simulink model "sedemo_star_routing"  (Simulink 7.5)
settings: Solver=VariableStepDiscrete  StartTime=0.0  StopTime=100  MaxStep=inf  RelTol=1e-3
undefined symbols (not defined in the file or in its folder): des_attributefunction_support
libraries: simeventsattributes2 x13, simeventssink1 x6, simeventsserver1 x5, simeventsrouting1 x4, simeventsgenerators1 x3, simeventstranslate1 x2, simeventsinfo x1
settings Model: Creator=The MathWorks Inc.  ExtModeAutoUpdateStatusClock=off
settings DataIOCC: SaveOutput=off  SignalLogging=off  SaveTime=off
settings OptimizationCC: InlineParams=on  InitFltsAndDblsToZero=on
settings DebuggingCC: AlgebraicLoopMsg=error  SolverPrmCheckMsg=none  StrictBusMsg=Warning
settings SimEventsCC: propDiagAttribOutput=1  propDiagFcnCallOutput=1  propDiagStatOutput=0

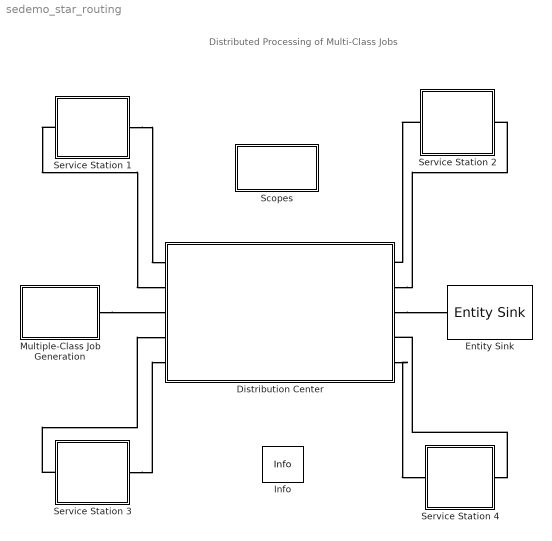
== system sedemo_star_routing ==
  note: Distributed Processing of Multi-Class Jobs
  Distribution Center : Subsystem  mask(Distribution Center){JobIDInWatch=1, RoutingDelay=.3}
      mask prompts: JobIDInWatch "Display service history for jobs with ID:"; RoutingDelay "Time needed for routing:"
      mask help:
      | Distribution center receives jobs from the source or remote service stations. It routes the job to its next service station based on job class and job service status.
      | Specify the time required for routing and the job ID that the service history monitor is tracing.
      mask Display:
      | color('blue')
      | fprintf('JOB ID: %s\n\nDouble Click to \nSelect Job ID.', get_param(gcb,'JobIDInWatch'))
  Entity Sink : simeventssink1/Entity Sink  Priority=1  SystemSampleTime=-1  AvailableForArrivals=on  StatNumberArrived=Off
  Info : simeventsinfo/Info  SystemSampleTime=-1
  Multiple-Class Job Generation : Subsystem
  Scopes : Subsystem
      mask Display: fprintf('Scopes')
  Service Station 1 : Subsystem
  Service Station 2 : Subsystem
  Service Station 3 : Subsystem
  Service Station 4 : Subsystem
  connections:
  Service Station 1/LConn1 -- Distribution Center/LConn2
  Distribution Center/RConn2 -- Service Station 2/LConn1
  Distribution Center/RConn5 -- Service Station 4/LConn1
  Service Station 3/LConn1 -- Distribution Center/LConn5
  Multiple-Class Job Generation/RConn1 -- Distribution Center/LConn3
  Distribution Center/RConn3 -- Entity Sink/LConn1
  Service Station 2/RConn1 -- Distribution Center/RConn1
  Service Station 1/RConn1 -- Distribution Center/LConn1
  Service Station 3/RConn1 -- Distribution Center/LConn4
  Service Station 4/RConn1 -- Distribution Center/RConn4

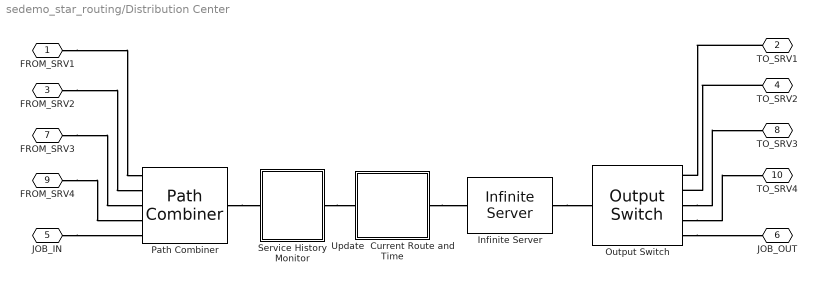
== system sedemo_star_routing/Distribution Center ==
  Infinite Server : simeventsserver1/Infinite Server  Priority=1  SystemSampleTime=-1  ServiceTimeFrom=Dialog  ServiceTime=RoutingDelay  AttributeName=ServiceTime  PriorityServiceCompletion=5  EnableTOPort=off  StatNumberDeparted=Off  StatNumberInBlock=Off  StatPendingEntity=Off  StatNumberPending=Off  StatAverageWait=Off  StatNumberTimedout=Off
  Output Switch : simeventsrouting1/Output Switch  Priority=1  SystemSampleTime=-1  NumberOutputPorts=5  SwitchingCriterion=From attribute  InitialSeed=34567  AttributeName=CurrentRoute  InitialConditionsOpt=off  InitialConditions=1  EntityBufferOpt=off  SpecifyEventPriority=off  PriorityOutputSwitchSelectPort=4100  TimeoutPortOpt=off  StatNumberDeparted=Off  StatNumberTimedOut=Off  StatPendingEntity=Off  StatLastDeparturePort=Off  EvaluatedNumPorts=5
  Path Combiner : simeventsrouting1/Path Combiner  Priority=1  SystemSampleTime=-1  NumberInputPorts=5  InputPortPrecedence=IN1 port  InitialSeed=45675  SpecifyEventPriority=off  PriorityPathCombinerPortPrecedenceSelection=4100  StatNumberDeparted=Off  StatLastArrivalPort=Off  EvaluatedNumPorts=5
  Service History Monitor : Subsystem
  Update  Current Route and Time : Subsystem  LoadFcn=des_attributefunction_support(gcb,'LoadFcn');  StartFcn=des_attributefunction_support(gcb,'StartFcn');  mask(Attribute Function){OutputNamePrefix=out_}
      mask prompts: OutputNamePrefix "Prefix name"
      settings: CopyFcn=des_attributefunction_support(gcb,'CopyFcn');  OpenFcn=des_attributefunction_support(gcb,'OpenFcn');  ErrorFcn=des_error_redirect
      mask Display: image(des_iconLoad('attribFunction.jpg'),'center');
  FROM_SRV1 : PMIOPort  Port=1  Side=Left
  TO_SRV1 : PMIOPort  Port=2  Side=Left
  FROM_SRV2 : PMIOPort  Port=3  Side=Right
  TO_SRV2 : PMIOPort  Port=4  Side=Right
  JOB_IN : PMIOPort  Port=5  Side=Left
  JOB_OUT : PMIOPort  Port=6  Side=Right
  FROM_SRV3 : PMIOPort  Port=7  Side=Left
  TO_SRV3 : PMIOPort  Port=8  Side=Left
  FROM_SRV4 : PMIOPort  Port=9  Side=Right
  TO_SRV4 : PMIOPort  Port=10  Side=Right
  connections:
  TO_SRV1/RConn1 -- Output Switch/RConn1
  FROM_SRV1/RConn1 -- Path Combiner/LConn1
  TO_SRV2/RConn1 -- Output Switch/RConn2
  FROM_SRV2/RConn1 -- Path Combiner/LConn2
  Output Switch/RConn3 -- TO_SRV3/RConn1
  Output Switch/RConn4 -- TO_SRV4/RConn1
  Output Switch/RConn5 -- JOB_OUT/RConn1
  FROM_SRV3/RConn1 -- Path Combiner/LConn3
  FROM_SRV4/RConn1 -- Path Combiner/LConn4
  JOB_IN/RConn1 -- Path Combiner/LConn5
  Path Combiner/RConn1 -- Service History Monitor/LConn1
  Update  Current Route and Time/RConn1 -- Infinite Server/LConn1
  Infinite Server/RConn1 -- Output Switch/LConn1
  Service History Monitor/RConn1 -- Update  Current Route and Time/LConn1

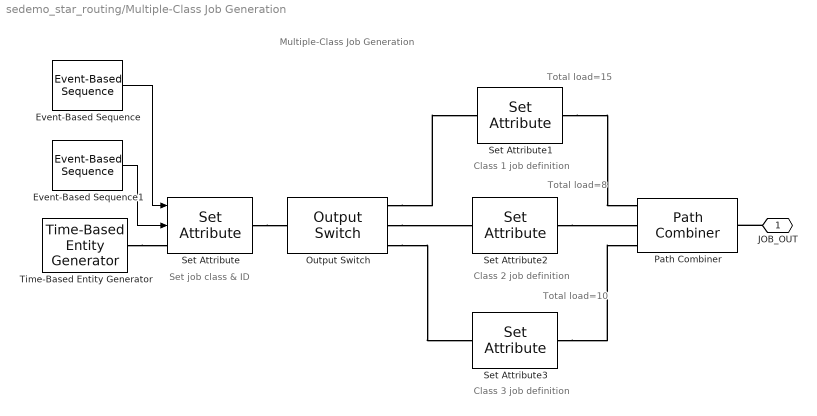
== system sedemo_star_routing/Multiple-Class Job Generation ==
  note: Set job class & ID
  note: Class 1 job definition
  note: Class 2 job definition
  note: Class 3 job definition
  note: Total load=15
  note: Total load=8
  note: Total load=10
  note: Multiple-Class Job Generation
  Event-Based Sequence : simeventsgenerators1/Signal Generators/Event-Based Sequence  SystemSampleTime=-1  VectorOutputValues=1:3  FormOutputOpt=Cyclic repetition  IsProcessed=on  isConnected=1
  Event-Based Sequence1 : simeventsgenerators1/Signal Generators/Event-Based Sequence  SystemSampleTime=-1  VectorOutputValues=1:15  FormOutputOpt=Cyclic repetition  IsProcessed=on  isConnected=1
  Output Switch : simeventsrouting1/Output Switch  Priority=1  SystemSampleTime=-1  NumberOutputPorts=3  SwitchingCriterion=From attribute  InitialSeed=34567  AttributeName=JobClass  InitialConditionsOpt=off  InitialConditions=1  EntityBufferOpt=off  SpecifyEventPriority=off  PriorityOutputSwitchSelectPort=4100  TimeoutPortOpt=off  StatNumberDeparted=Off  StatNumberTimedOut=Off  StatPendingEntity=Off  StatLastDeparturePort=Off  EvaluatedNumPorts=3
  Path Combiner : simeventsrouting1/Path Combiner  Priority=1  SystemSampleTime=-1  NumberInputPorts=3  InputPortPrecedence=IN1 port  InitialSeed=45675  SpecifyEventPriority=off  PriorityPathCombinerPortPrecedenceSelection=4100  StatNumberDeparted=Off  StatLastArrivalPort=Off  EvaluatedNumPorts=3
  Set Attribute : simeventsattributes2/Set Attribute  Priority=1  DialogController=des_ddg_create  DialogControllerArgs=DataTag19  SystemSampleTime=-1  AttributeFrom=Signal port|Signal port|Dialog|Dialog  AttributeName=JobClass|JobID|LastServiceLocation|JobServiceStatus  AttributeTreatAsVector=1|1|1|0  AttributeValue=1|1|0|zeros(1,15)  AttributeCreate=on  StatNumberDeparted=Off  EvaluatedAttributeValue={1}
  Set Attribute1 : simeventsattributes2/Set Attribute  Priority=1  DialogController=des_ddg_create  DialogControllerArgs=DataTag21  SystemSampleTime=-1  AttributeFrom=Dialog|Dialog|Dialog  AttributeName=ServiceProcess|ServiceTime|CurrentStep  AttributeTreatAsVector=1|1|1  AttributeValue=[1 2 4 2 3 5]|[2 1 5 3 4 0]|1  AttributeCreate=on  StatNumberDeparted=Off  EvaluatedAttributeValue={1}
  Set Attribute2 : simeventsattributes2/Set Attribute  Priority=1  DialogController=des_ddg_create  DialogControllerArgs=DataTag23  SystemSampleTime=-1  AttributeFrom=Dialog|Dialog|Dialog  AttributeName=ServiceProcess|ServiceTime|CurrentStep  AttributeTreatAsVector=1|1|1  AttributeValue=[2 1 3 1 4 5]|[1 1 2 1 3 0]|1  AttributeCreate=on  StatNumberDeparted=Off  EvaluatedAttributeValue={1}
  Set Attribute3 : simeventsattributes2/Set Attribute  Priority=1  DialogController=des_ddg_create  DialogControllerArgs=DataTag25  SystemSampleTime=-1  AttributeFrom=Dialog|Dialog|Dialog  AttributeName=ServiceProcess|ServiceTime|CurrentStep  AttributeTreatAsVector=1|1|1  AttributeValue=[4 2 1 2 3 5]|[5 1 2 1 1 0]|1  AttributeCreate=on  StatNumberDeparted=Off  EvaluatedAttributeValue={1}
  Time-Based Entity Generator : simeventsgenerators1/Entity Generators/Time-Based Entity Generator  Priority=1  DialogController=des_ddg_create  DialogControllerArgs=DataTag27  SystemSampleTime=-1  GenerateEntitiesUpon=Intergeneration time from dialog  Distribution=Uniform  Minimum=1  Maximum=2  Mean=1  InitialSeed=12345  Period=1  PriorityEntityGeneration=600  GenerateEntityAtSimulationStart=on  ResponseWhenBlocked=Pause generation  ResponseWhenUnblocked=Immediate restart  EntityType=Blank  StatNumberDeparted=Off  StatPendingEntity=Off  StatAverageIntergenerationTime=Off
  JOB_OUT : PMIOPort  Port=1  Side=Right
  wires:
  Event-Based Sequence/1 -> Set Attribute/1
  Event-Based Sequence1/1 -> Set Attribute/2
  connections:
  Set Attribute/RConn1 -- Output Switch/LConn1
  Output Switch/RConn1 -- Set Attribute1/LConn1
  Output Switch/RConn2 -- Set Attribute2/LConn1
  Output Switch/RConn3 -- Set Attribute3/LConn1
  Set Attribute1/RConn1 -- Path Combiner/LConn1
  Set Attribute2/RConn1 -- Path Combiner/LConn2
  Set Attribute3/RConn1 -- Path Combiner/LConn3
  Time-Based Entity Generator/RConn1 -- Set Attribute/LConn1
  JOB_OUT/RConn1 -- Path Combiner/RConn1

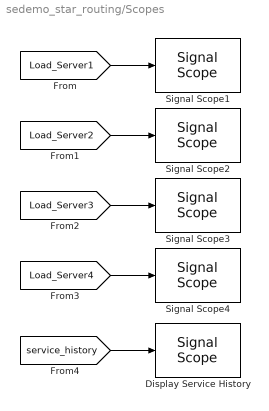
== system sedemo_star_routing/Scopes ==
  Display Service History : simeventssink1/Signal Scope  Priority=1  SystemSampleTime=-1  PlotType=Stair  InputType=Signal  NumInputs=1  AttributeNameY=Count  XInputOptionSignal=Event time  XInputOptionEntity=Event time  AttributeNameX=Count  EnableEntityOutport=on  XMin=0  XMax=110  XLimitExceededOption=Keep axis limits unchanged  YLimitExceededOption=Keep axis limits unchanged  AxisGrid=on  AxisLegend=off  LineDisables=""  LineColors="0  0  1"  LineStyles=-  LineMarkers=None  OpenScopeAtSimStart=on  Title=Service History for Jobs with Specified ID  YLabel=Service Station Visited  XLabel=Time  FigurePosition=[7 687 320 160]  AxisZoom=off  DataStoreOption=Limited  DataPointsLimit=10000  StatNumberArrived=Off  ShowCountPlotted=off  ShowToolbar=off
      settings: YMin=0  YMax=5
  Signal Scope1 : simeventssink1/Signal Scope  Priority=1  SystemSampleTime=-1  PlotType=Stair  InputType=Signal  NumInputs=1  AttributeNameY=Count  XInputOptionSignal=Event time  XInputOptionEntity=Event time  AttributeNameX=Count  EnableEntityOutport=on  XMin=0  XMax=10  XLimitExceededOption=Stretch axis limits  YLimitExceededOption=Stretch axis limits  AxisGrid=on  AxisLegend=off  LineDisables=""  LineColors="0  0  1"  LineStyles=-  LineMarkers=.  OpenScopeAtSimStart=on  Title=Load of Service Station 1  YLabel=Load  XLabel=Time  FigurePosition=[6 499 314 139]  AxisZoom=off  DataStoreOption=Limited  DataPointsLimit=10000  StatNumberArrived=Off  ShowCountPlotted=off  ShowToolbar=off
      settings: YMin=0  YMax=6
  Signal Scope2 : simeventssink1/Signal Scope  Priority=1  SystemSampleTime=-1  PlotType=Stair  InputType=Signal  NumInputs=1  AttributeNameY=Count  XInputOptionSignal=Event time  XInputOptionEntity=Event time  AttributeNameX=Count  EnableEntityOutport=on  XMin=0  XMax=10  XLimitExceededOption=Stretch axis limits  YLimitExceededOption=Stretch axis limits  AxisGrid=on  AxisLegend=off  LineDisables=""  LineColors="1  0  1"  LineStyles=-  LineMarkers=.  OpenScopeAtSimStart=on  Title=Load of Service Station 2  YLabel=Load  XLabel=Time  FigurePosition=[328 499 314 140]  AxisZoom=off  DataStoreOption=Limited  DataPointsLimit=10000  StatNumberArrived=Off  ShowCountPlotted=off  ShowToolbar=off
      settings: YMin=0  YMax=6
  Signal Scope3 : simeventssink1/Signal Scope  Priority=1  SystemSampleTime=-1  PlotType=Stair  InputType=Signal  NumInputs=1  AttributeNameY=Count  XInputOptionSignal=Event time  XInputOptionEntity=Event time  AttributeNameX=Count  EnableEntityOutport=on  XMin=0  XMax=10  XLimitExceededOption=Stretch axis limits  YLimitExceededOption=Stretch axis limits  AxisGrid=on  AxisLegend=off  LineDisables=""  LineColors="0  1  0"  LineStyles=-  LineMarkers=.  OpenScopeAtSimStart=on  Title=Load of Service Station 3  YLabel=Load  XLabel=Time  FigurePosition=[5 314 314 137]  AxisZoom=off  DataStoreOption=Limited  DataPointsLimit=10000  StatNumberArrived=Off  ShowCountPlotted=off  ShowToolbar=off
      settings: YMin=0  YMax=6
  Signal Scope4 : simeventssink1/Signal Scope  Priority=1  SystemSampleTime=-1  PlotType=Stair  InputType=Signal  NumInputs=1  AttributeNameY=Count  XInputOptionSignal=Event time  XInputOptionEntity=Event time  AttributeNameX=Count  EnableEntityOutport=on  XMin=0  XMax=10  XLimitExceededOption=Stretch axis limits  YLimitExceededOption=Stretch axis limits  AxisGrid=on  AxisLegend=off  LineDisables=""  LineColors="1  0  0"  LineStyles=-  LineMarkers=.  OpenScopeAtSimStart=on  Title=Load of Service Station 4  YLabel=Load  XLabel=Time  FigurePosition=[328 316 318 134]  AxisZoom=off  DataStoreOption=Limited  DataPointsLimit=10000  StatNumberArrived=Off  ShowCountPlotted=off  ShowToolbar=off
      settings: YMin=0  YMax=6
  wires:
  [Load_Server1] -> Signal Scope1/1
  [Load_Server4] -> Signal Scope4/1
  [Load_Server3] -> Signal Scope3/1
  [Load_Server2] -> Signal Scope2/1
  [service_history] -> Display Service History/1

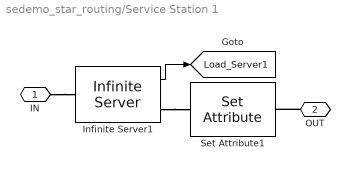
== system sedemo_star_routing/Service Station 1 ==
  Infinite Server1 : simeventsserver1/Infinite Server  Priority=1  SystemSampleTime=-1  ServiceTimeFrom=Attribute  ServiceTime=1  AttributeName=CurrentServiceTime  PriorityServiceCompletion=500  EnableTOPort=off  StatNumberDeparted=Off  StatNumberInBlock=On  StatPendingEntity=Off  StatNumberPending=Off  StatAverageWait=Off  StatNumberTimedout=Off
  Set Attribute1 : simeventsattributes2/Set Attribute  Priority=1  DialogController=des_ddg_create  DialogControllerArgs=DataTag35  SystemSampleTime=-1  AttributeFrom=Dialog  AttributeName=LastServiceLocation  AttributeTreatAsVector=1  AttributeValue=1  AttributeCreate=on  StatNumberDeparted=Off  EvaluatedAttributeValue={1}
  IN : PMIOPort  Port=1  Side=Left
  OUT : PMIOPort  Port=2  Side=Right
  tag scope: Load_Server1=global
  wires:
  Infinite Server1/1 -> [Load_Server1]
  connections:
  Infinite Server1/RConn1 -- Set Attribute1/LConn1
  IN/RConn1 -- Infinite Server1/LConn1
  OUT/RConn1 -- Set Attribute1/RConn1

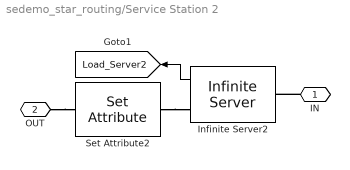
== system sedemo_star_routing/Service Station 2 ==
  Infinite Server2 : simeventsserver1/Infinite Server  Priority=1  SystemSampleTime=-1  ServiceTimeFrom=Attribute  ServiceTime=1  AttributeName=CurrentServiceTime  PriorityServiceCompletion=500  EnableTOPort=off  StatNumberDeparted=Off  StatNumberInBlock=On  StatPendingEntity=Off  StatNumberPending=Off  StatAverageWait=Off  StatNumberTimedout=Off
  Set Attribute2 : simeventsattributes2/Set Attribute  Priority=1  DialogController=des_ddg_create  DialogControllerArgs=DataTag38  SystemSampleTime=-1  AttributeFrom=Dialog  AttributeName=LastServiceLocation  AttributeTreatAsVector=1  AttributeValue=2  AttributeCreate=on  StatNumberDeparted=Off  EvaluatedAttributeValue={2}
  IN : PMIOPort  Port=1  Side=Left
  OUT : PMIOPort  Port=2  Side=Right
  tag scope: Load_Server2=global
  wires:
  Infinite Server2/1 -> [Load_Server2]
  connections:
  Set Attribute2/LConn1 -- Infinite Server2/RConn1
  IN/RConn1 -- Infinite Server2/LConn1
  OUT/RConn1 -- Set Attribute2/RConn1

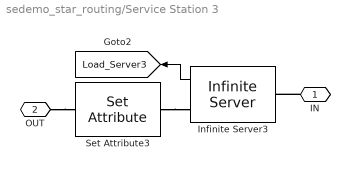
== system sedemo_star_routing/Service Station 3 ==
  Infinite Server3 : simeventsserver1/Infinite Server  Priority=1  SystemSampleTime=-1  ServiceTimeFrom=Attribute  ServiceTime=1  AttributeName=CurrentServiceTime  PriorityServiceCompletion=500  EnableTOPort=off  StatNumberDeparted=Off  StatNumberInBlock=On  StatPendingEntity=Off  StatNumberPending=Off  StatAverageWait=Off  StatNumberTimedout=Off
  Set Attribute3 : simeventsattributes2/Set Attribute  Priority=1  DialogController=des_ddg_create  DialogControllerArgs=DataTag41  SystemSampleTime=-1  AttributeFrom=Dialog  AttributeName=LastServiceLocation  AttributeTreatAsVector=1  AttributeValue=3  AttributeCreate=on  StatNumberDeparted=Off  EvaluatedAttributeValue={3}
  IN : PMIOPort  Port=1  Side=Left
  OUT : PMIOPort  Port=2  Side=Right
  tag scope: Load_Server3=global
  wires:
  Infinite Server3/1 -> [Load_Server3]
  connections:
  Set Attribute3/LConn1 -- Infinite Server3/RConn1
  IN/RConn1 -- Infinite Server3/LConn1
  OUT/RConn1 -- Set Attribute3/RConn1

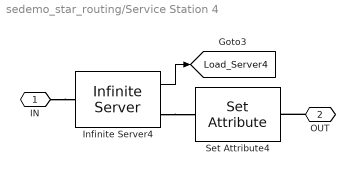
== system sedemo_star_routing/Service Station 4 ==
  Infinite Server4 : simeventsserver1/Infinite Server  Priority=1  SystemSampleTime=-1  ServiceTimeFrom=Attribute  ServiceTime=1  AttributeName=CurrentServiceTime  PriorityServiceCompletion=500  EnableTOPort=off  StatNumberDeparted=Off  StatNumberInBlock=On  StatPendingEntity=Off  StatNumberPending=Off  StatAverageWait=Off  StatNumberTimedout=Off
  Set Attribute4 : simeventsattributes2/Set Attribute  Priority=1  DialogController=des_ddg_create  DialogControllerArgs=DataTag44  SystemSampleTime=-1  AttributeFrom=Dialog  AttributeName=LastServiceLocation  AttributeTreatAsVector=1  AttributeValue=4  AttributeCreate=on  StatNumberDeparted=Off  EvaluatedAttributeValue={4}
  IN : PMIOPort  Port=1  Side=Left
  OUT : PMIOPort  Port=2  Side=Right
  tag scope: Load_Server4=global
  wires:
  Infinite Server4/1 -> [Load_Server4]
  connections:
  Infinite Server4/RConn1 -- Set Attribute4/LConn1
  IN/RConn1 -- Infinite Server4/LConn1
  OUT/RConn1 -- Set Attribute4/RConn1

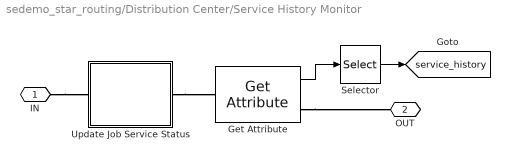
== system sedemo_star_routing/Distribution Center/Service History Monitor ==
  Get Attribute : simeventsattributes2/Get Attribute  Priority=1  DialogController=des_ddg_create  DialogControllerArgs=DataTag4  SystemSampleTime=-1  AttributeName=JobServiceStatus  AttributeMissing=Error  AttributeDefaultValue=1  AttributeSendTiming=After entity departure  AttributeTreatAsVector=1  StatNumberDeparted=Off
  Selector : Selector  InputPortWidth=15  IndexOptions=Index vector (dialog)  Indices=[JobIDInWatch]  OutputSizes=1
  Update Job Service Status : Subsystem  LoadFcn=des_attributefunction_support(gcb,'LoadFcn');  StartFcn=des_attributefunction_support(gcb,'StartFcn');  mask(Attribute Function){OutputNamePrefix=out_}
      mask prompts: OutputNamePrefix "Prefix name"
      settings: CopyFcn=des_attributefunction_support(gcb,'CopyFcn');  OpenFcn=des_attributefunction_support(gcb,'OpenFcn');  ErrorFcn=des_error_redirect
      mask Display: image(des_iconLoad('attribFunction.jpg'),'center');
  IN : PMIOPort  Port=1  Side=Left
  OUT : PMIOPort  Port=2  Side=Right
  tag scope: service_history=global
  wires:
  Get Attribute/1 -> Selector/1
  Selector/1 -> [service_history]
  connections:
  IN/RConn1 -- Update Job Service Status/LConn1
  Get Attribute/RConn1 -- OUT/RConn1
  Update Job Service Status/RConn1 -- Get Attribute/LConn1

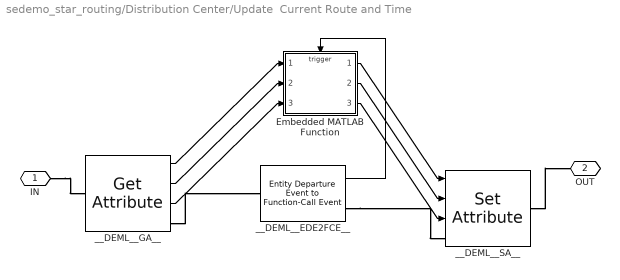
== system sedemo_star_routing/Distribution Center/Update  Current Route and Time ==
  Embedded MATLAB Function : Stateflow chart  TreatAsAtomicUnit=on
      settings: PropExecContextOutsideSubsystem=on
  __DEML__EDE2FCE__ : simeventstranslate1/Entity Departure Event to Function-Call Event  Priority=1  SystemSampleTime=-1  TimingFunctionCallF1=Before entity departure  EnableE1Port=off  EnableF2Port=off  TimingFunctionCallF2=Before entity departure  EnableE2Port=off  StatNumberDeparted=Off  StatNumberF1Calls=Off  StatNumberF2Calls=Off  IsInsideAFB=on
  __DEML__GA__ : simeventsattributes2/Get Attribute  Priority=1  DialogController=des_ddg_create  DialogControllerArgs=DataTag12  SystemSampleTime=-1  AttributeName=ServiceProcess|ServiceTime|CurrentStep  AttributeMissing=Error|Error|Error  AttributeDefaultValue=1|1|1  AttributeSendTiming=Before entity departure|Before entity departure|Before entity departure  AttributeTreatAsVector=1|1|1  StatNumberDeparted=Off  EvaluatedDefaultAttributeValue={[];[];[]}
  __DEML__SA__ : simeventsattributes2/Set Attribute  Priority=1  DialogController=des_ddg_create  DialogControllerArgs=DataTag14  SystemSampleTime=-1  AttributeFrom=Signal port|Signal port|Signal port  AttributeName=CurrentRoute|CurrentServiceTime|CurrentStep  AttributeTreatAsVector=1|1|1  AttributeValue=1|1|1  AttributeCreate=on  StatNumberDeparted=Off  EvaluatedAttributeValue={[];[];[]}
  IN : PMIOPort  Port=1  Side=Left
  OUT : PMIOPort  Port=2  Side=Right
  wires:
  __DEML__EDE2FCE__/1 -> Embedded MATLAB Function/Trigger
  __DEML__GA__/1 -> Embedded MATLAB Function/1(ServiceProcess)
  __DEML__GA__/2 -> Embedded MATLAB Function/2(ServiceTime)
  __DEML__GA__/3 -> Embedded MATLAB Function/3(CurrentStep)
  Embedded MATLAB Function/1(out_CurrentRoute) -> __DEML__SA__/1
  Embedded MATLAB Function/2(out_CurrentServiceTime) -> __DEML__SA__/2
  Embedded MATLAB Function/3(out_CurrentStep) -> __DEML__SA__/3
  connections:
  __DEML__SA__/RConn1 -- OUT/RConn1
  IN/RConn1 -- __DEML__GA__/LConn1
  __DEML__GA__/RConn1 -- __DEML__EDE2FCE__/LConn1
  __DEML__EDE2FCE__/RConn1 -- __DEML__SA__/LConn1

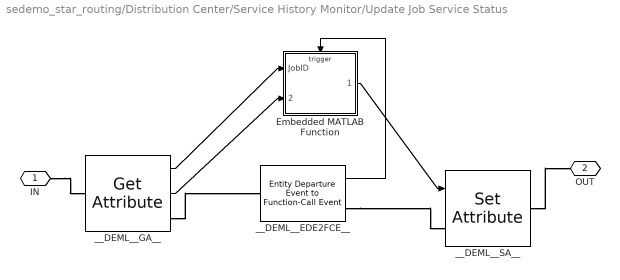
== system sedemo_star_routing/Distribution Center/Service History Monitor/Update Job Service Status ==
  Embedded MATLAB Function : Stateflow chart  TreatAsAtomicUnit=on
      settings: PropExecContextOutsideSubsystem=on
  __DEML__EDE2FCE__ : simeventstranslate1/Entity Departure Event to Function-Call Event  Priority=1  SystemSampleTime=-1  TimingFunctionCallF1=Before entity departure  EnableE1Port=off  EnableF2Port=off  TimingFunctionCallF2=Before entity departure  EnableE2Port=off  StatNumberDeparted=Off  StatNumberF1Calls=Off  StatNumberF2Calls=Off  IsInsideAFB=on
  __DEML__GA__ : simeventsattributes2/Get Attribute  Priority=1  DialogController=des_ddg_create  DialogControllerArgs=DataTag7  SystemSampleTime=-1  AttributeName=JobID|LastServiceLocation  AttributeMissing=Error|Error  AttributeDefaultValue=1|1  AttributeSendTiming=Before entity departure|Before entity departure  AttributeTreatAsVector=1|1  StatNumberDeparted=Off  EvaluatedDefaultAttributeValue={[];[]}
  __DEML__SA__ : simeventsattributes2/Set Attribute  Priority=1  DialogController=des_ddg_create  DialogControllerArgs=DataTag9  SystemSampleTime=-1  AttributeFrom=Signal port  AttributeName=JobServiceStatus  AttributeTreatAsVector=1  AttributeValue=1  AttributeCreate=on  StatNumberDeparted=Off  EvaluatedAttributeValue={[]}
  IN : PMIOPort  Port=1  Side=Left
  OUT : PMIOPort  Port=2  Side=Right
  wires:
  __DEML__EDE2FCE__/1 -> Embedded MATLAB Function/Trigger
  __DEML__GA__/1 -> Embedded MATLAB Function/1(JobID)
  __DEML__GA__/2 -> Embedded MATLAB Function/2(LastServiceLocation)
  Embedded MATLAB Function/1(out_JobServiceStatus) -> __DEML__SA__/1
  connections:
  __DEML__EDE2FCE__/RConn1 -- __DEML__SA__/LConn1
  __DEML__GA__/RConn1 -- __DEML__EDE2FCE__/LConn1
  IN/RConn1 -- __DEML__GA__/LConn1
  __DEML__SA__/RConn1 -- OUT/RConn1

== matlab function Distribution Center/Update Current Route and Time/Embedded MATLAB Function ==
  data: ServiceProcess input double; out_CurrentRoute output double; out_CurrentServiceTime output double; ServiceTime input double; CurrentStep input double; out_CurrentStep output double
  events: trigger input FUNCTION_CALL_EVENT
function [out_CurrentRoute, out_CurrentServiceTime, out_CurrentStep] ...
    = fcn(ServiceProcess, ServiceTime, CurrentStep)
% This function defines the routing logic of the distribution center. 
% It uses CurrentStep to index into ServiceProcess to choose the next 
% CurrentRoute for the job.  It also indexes into ServiceTime to choose
% the next CurrentServiceTime for the job.

out_CurrentRoute = ServiceProcess(CurrentStep);
out_CurrentServiceTime = ServiceTime(CurrentStep);
out_CurrentStep = CurrentStep + 1;

== matlab function Distribution Center/Service History Monitor/Update Job Service Status/Embedded MATLAB Function ==
  data: JobID input double; out_JobServiceStatus output double; LastServiceLocation input double
  events: trigger input FUNCTION_CALL_EVENT
function out_JobServiceStatus = fcn(JobID,LastServiceLocation)
% This function uses a Embedded MATLAB persistent variable to
% trace the service history of jobs. When an entity representing
% a job passes this block, the function detects the job ID and 
% its last service location and updates the service history of this 
% job. The service history data is then carried by the passing entity
% for instrumentation purpose.

persistent curServiceHistory;

if isempty(curServiceHistory)
    curServiceHistory = repmat(NaN,1,15);
end

curServiceHistory(JobID) = LastServiceLocation;

out_JobServiceStatus = curServiceHistory;
